simulink model "ksp_zad19_ms"  (Simulink 2.20)
settings: Solver=ode45  StartTime=0.0  StopTime=200  MaxStep=0.10  RelTol=1e-3  AbsTol=1e-6
values from neighbouring files (symbols this model uses):
  D = fp(3)    [pidfunc.m]
  I = fp(2)    [pidfunc.m]
  P = fp(1)    [pidfunc.m]
libraries: PID_continous_block x1
settings Model: InitialStep=0.10  ConsistencyChecking=off  RTWPlaceOutputsASAP=off

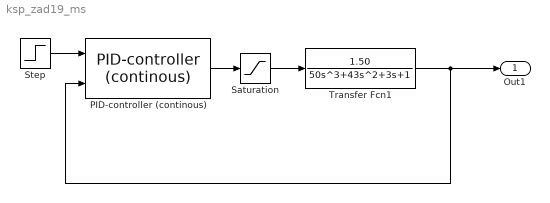
== system ksp_zad19_ms ==
  PID-controller (continous) : PID_continous_block/PID-controller (continous)  Description=PID_regulator  P=P  I=I  D=D
  Saturation : Saturate  UpperLimit=10  LowerLimit=0
  Step : Step  Time=0  Before=0  After=1
  Transfer Fcn1 : TransferFcn  Numerator=[1.50]  Denominator=[50 43 3 1]
  Out1 : Outport  Port=1
  wires:
  Step/1 -> PID-controller (continous)/1
  Transfer Fcn1/1 -> Out1/1, PID-controller (continous)/2
  Saturation/1 -> Transfer Fcn1/1
  PID-controller (continous)/1 -> Saturation/1
